simulink model "Coding_Matrix_Test1"  (R2021a)
settings: Solver=VariableStepAuto  StartTime=0.0  StopTime=100  FixedStep=0.1  RelTol=1e-3
values from neighbouring files (symbols this model uses):
  sample_time = 1    [main1.m]    (also in main2.m)
undefined symbols (not defined in the file or in its folder): Discrete, Time
libraries: dspsrcs4 x1, ctrlSharedLib x1
settings Model: Creator=mehra  LastModifiedBy=mehra

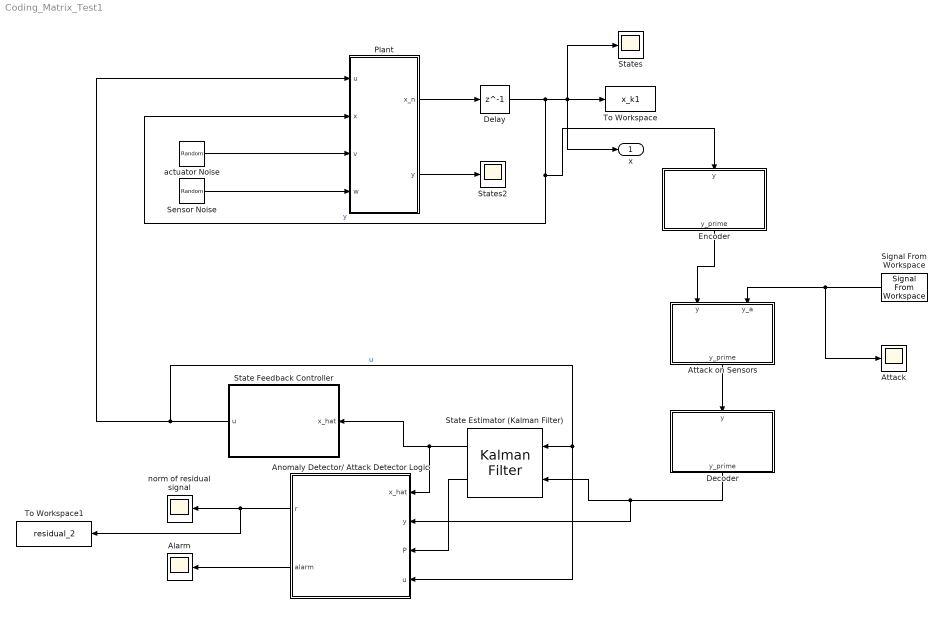
== system Coding_Matrix_Test1 ==
  Alarm : Scope
  Anomaly Detector/ Attack Detector Logic : MATLAB Function  TreatAsAtomicUnit=on
  Attack : Scope
  Attack on Sensors : MATLAB Function  TreatAsAtomicUnit=on
  Decoder : MATLAB Function  TreatAsAtomicUnit=on
  Delay : Delay  DelayLength=1  InitialCondition=[0;0]  SampleTime=sample_time
  Encoder : MATLAB Function  TreatAsAtomicUnit=on
  Plant : MATLAB Function  TreatAsAtomicUnit=on
  Sensor Noise : RandomNumber  Mean=[0 0]  Variance=[0.01 0.01]  Seed=[randi(100) randi(100)]  SampleTime=sample_time
  Signal From Workspace : dspsrcs4/Signal From Workspace  X=y_a  Ts=sample_time  nsamps=1  OutputAfterFinalValue=Cyclic repetition  ignoreOrWarnInputAndFrameLengths=off  OutputFrames=off
  State Estimator (Kalman Filter) : ctrlSharedLib/Kalman Filter  TimeDomain=Discrete-Time  UseCurrentEstimator=on  ModelSource=Individual A, B, C, D matrices  ModelSourceVariable=ss(0.95,1,1,0,1)  A=[0.8 0; 0.5 1]  B=[1;0.5]  C=[2 0.5;0 1]  D=0  NumberOfStates=1  NumberOfInputs=1  NumberOfOutputs=1  InitialEstimateSource=Dialog  X0=[0 0]'  P0=10  UseK=off  UseGH=off  NumberOfProcessNoiseInputs=1  G=1  TimeInvariantG=on  H=0  TimeInvariantH=on  Q=0.001  TimeInvariantQ=on  R=0.001  TimeInvariantR=on  N=0  TimeInvariantN=on  AddInputPort=on  AddEnablePort=off  OutputEstimatedY=off  OutputP=on  Ts=sample_time
  State Feedback Controller : MATLAB Function  TreatAsAtomicUnit=on
  States : Scope
  States2 : Scope
  To Workspace : ToWorkspace  VariableName=x_k1  SaveFormat=Timeseries  SampleTime=sample_time
  To Workspace1 : ToWorkspace  VariableName=residual_2  SaveFormat=Timeseries  SampleTime=sample_time
  actuator Noise : RandomNumber  Mean=[0 0]  Variance=[0.0001 0.0001]  Seed=[randi(100) randi(100)]  SampleTime=sample_time
  norm of residual signal : Scope
  "x " : Outport  VectorParamsAs1DForOutWhenUnconnected=off
  wires:
  Plant/1(x_n) -> Delay/1
  actuator Noise/1 -> Plant/3(v)
  Sensor Noise/1 -> Plant/4(w)
  Delay/1 -> "x "/1, States/1, To Workspace/1, Plant/2(x), Encoder/1(y)  "y"
  Plant/2(y) -> States2/1
  Anomaly Detector/ Attack Detector Logic/1(r) -> To Workspace1/1, norm of residual signal/1
  Attack on Sensors/1(y_prime) -> Decoder/1(y)
  Encoder/1(y_prime) -> Attack on Sensors/1(y)
  Decoder/1(y_prime) -> Anomaly Detector/ Attack Detector Logic/2(y), State Estimator (Kalman Filter)/2
  Signal From Workspace/1 -> Attack/1, Attack on Sensors/2(y_a)
  Anomaly Detector/ Attack Detector Logic/2(alarm) -> Alarm/1
  State Estimator (Kalman Filter)/1 -> Anomaly Detector/ Attack Detector Logic/1(x_hat), State Feedback Controller/1(x_hat)
  State Feedback Controller/1(u) -> State Estimator (Kalman Filter)/1, Anomaly Detector/ Attack Detector Logic/4(u), Plant/1(u)  "u"
  State Estimator (Kalman Filter)/2 -> Anomaly Detector/ Attack Detector Logic/3(P)

== matlab function Coding_Matrix_Test1/Plant ==
  data: x_n output; u input; y output; x input; v input; w input
function [x_n, y] = fcn(u, x, v, w)

%A=[1.0000    0.0001   -0.0010;0.5747    1.0000   -0.0003;0.0162    0.0000    1.0000];
%B = [0.1   -0.2; -0.0536    0.0332;0.1955   -0.5294];

A = [0.8 0; 0.5 1];
B = [1;0.5];
C = [2 0.5;0 1];
D = 0;

x_n = A*x + B*u + v;
y = C*x + D*u + w;

== matlab function Coding_Matrix_Test1/Attack on Sensors ==
  data: y input; y_prime output; y_a input
function y_prime = fcn(y, y_a)
% this function should contain the attacker action on the sensor
% measurements
sigma1 = [2 -0.5;-0.5 1];
sigma2 = [1 -1;2 0];

y_prime = y_a';
% y_prime = y;

end

== matlab function Coding_Matrix_Test1/State Feedback Controller ==
  data: x_hat input; u output
function u  = Controller(x_hat)
%two tanks model 



K = [-1  -4];

u = K*x_hat;

== matlab function Coding_Matrix_Test1/Anomaly Detector// Attack Detector Logic ==
  data: x_hat input; y input; r output; P input; alarm output; u input
function [r, alarm] = Detector(x_hat,y, P, u)
% this function should contain the detection strategy

% for the chi square detector "P" should be the name of detection signal and
% "tau" the name of threshold
A = [0.8 0; 0.5 1];
B = [1;0.5];
C = [2 0.5;0 1];
threshold = chi2inv(0.99,2);
sigma = ((C)*(P)*(C')) + 0.01;
r = norm(y - C*(A*x_hat + B*u),2);
z = (r') * (inv(sigma)) * r;
if z<=threshold
    alarm = 0;
else
    alarm = 1;
end
alarm = alarm;
residual = z;
threshold = threshold;
end

== matlab function Coding_Matrix_Test1/Encoder ==
  data: y input; y_prime output
function y_prime = fcn(y)
% this function should contain the attacker action on the sensor
% measurements
sigma1 = [2 -0.5;-0.5 1];
sigma2 = [1 -1;2 0];
% y_prime = y'*sigma1;
y_prime = y;
end

== matlab function Coding_Matrix_Test1/Decoder ==
  data: y input; y_prime output
function y_prime = fcn(y)
% this function should contain the attacker action on the sensor
% measurements
sigma1 = [2 -0.5;-0.5 1];
sigma2 = [1 -1;2 0];
% y_prime = y*inv(sigma1);
y_prime = y;
end
